simulink library "ESTS_VVSO_WHL"  (R2022a)
settings: Solver=VariableStepAuto  StartTime=0.0  StopTime=10.0  RelTol=1e-3
libraries: ESTS_VVSO_WHL_LgtLoadTransf x1, ESTS_VVSO_WHL_LatLoadTransf x1
settings Model: Creator=blatak  LastModifiedBy=blatak

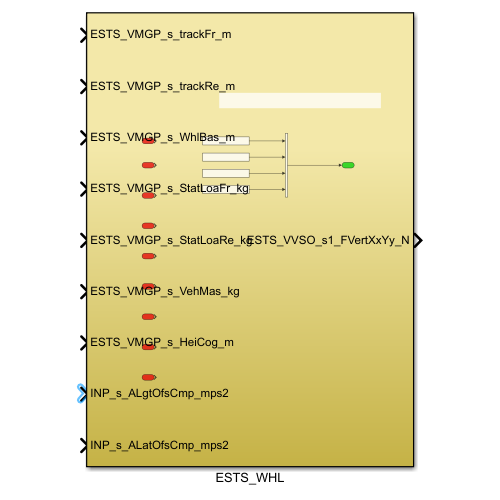
[thumbnail: Simulink's stored preview of the top-level diagram]
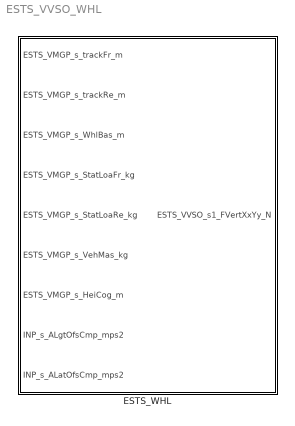
== system ESTS_VVSO_WHL ==
  ESTS_WHL : Subsystem

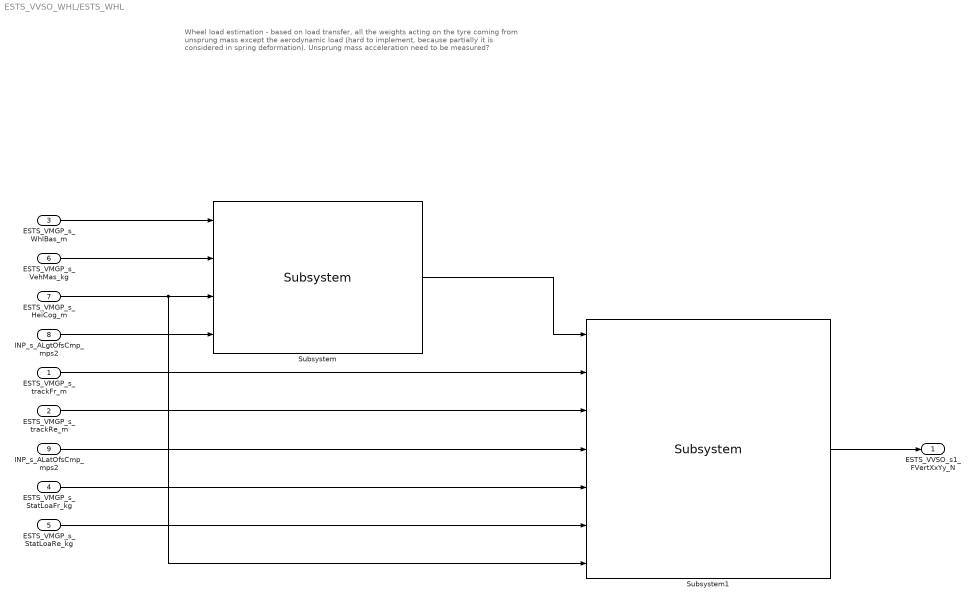
== system ESTS_VVSO_WHL/ESTS_WHL ==
  note: Wheel load estimation - based on load transfer, all the weights acting on the tyre coming
      | from unsprung mass except the aerodynamic load (hard to implement, because partially it is considered in spring deformation). Unsprung mass acceleration need to be measured?
  ESTS_VMGP_s_trackFr_m : Inport
  ESTS_VMGP_s_trackRe_m : Inport  Port=2
  ESTS_VMGP_s_WhlBas_m : Inport  Port=3
  ESTS_VMGP_s_StatLoaFr_kg : Inport  Port=4
  ESTS_VMGP_s_StatLoaRe_kg : Inport  Port=5
  ESTS_VMGP_s_VehMas_kg : Inport  Port=6
  ESTS_VMGP_s_HeiCog_m : Inport  Port=7
  INP_s_ALgtOfsCmp_mps2 : Inport  Port=8
  INP_s_ALatOfsCmp_mps2 : Inport  Port=9
  Subsystem : ESTS_VVSO_WHL_LgtLoadTransf/Subsystem  SystemSampleTime=-1  VariantActivationTime=update diagram  Latency=0  AutoFrameSizeCalculation=off
  Subsystem1 : ESTS_VVSO_WHL_LatLoadTransf/Subsystem  SystemSampleTime=-1  VariantActivationTime=update diagram  Latency=0  AutoFrameSizeCalculation=off
  ESTS_VVSO_s1_FVertXxYy_N : Outport
  wires:
  ESTS_VMGP_s_WhlBas_m/1 -> Subsystem/1
  ESTS_VMGP_s_VehMas_kg/1 -> Subsystem/2
  ESTS_VMGP_s_HeiCog_m/1 -> Subsystem1/7, Subsystem/3
  INP_s_ALgtOfsCmp_mps2/1 -> Subsystem/4
  Subsystem/1 -> Subsystem1/1
  ESTS_VMGP_s_trackFr_m/1 -> Subsystem1/2
  ESTS_VMGP_s_trackRe_m/1 -> Subsystem1/3
  INP_s_ALatOfsCmp_mps2/1 -> Subsystem1/4
  ESTS_VMGP_s_StatLoaFr_kg/1 -> Subsystem1/5
  ESTS_VMGP_s_StatLoaRe_kg/1 -> Subsystem1/6
  Subsystem1/1 -> ESTS_VVSO_s1_FVertXxYy_N/1
